simulink model "clutch_lockup"  (R2020b)
settings: Solver=VariableStepAuto  StartTime=0.0  StopTime=10.0  RelTol=1e-3
values from neighbouring files (symbols this model uses):
  be = 2.0    [initialization_data.sldd]
  bv = 1.0    [initialization_data.sldd]
  Ie = 1.0    [initialization_data.sldd]
  Iv = 5.0    [initialization_data.sldd]
  R = 1.0    [initialization_data.sldd]
  uk = 1.0    [initialization_data.sldd]
  us = 1.5    [initialization_data.sldd]
settings Model: Creator=Vrunda M Balgi  LastModifiedBy=Vrunda M Balgi

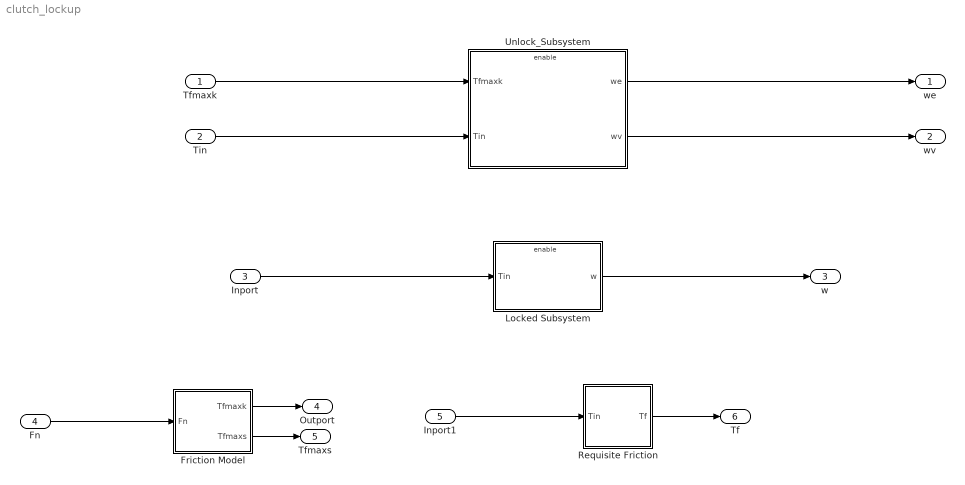
== system clutch_lockup ==
  Tfmaxk : Inport
  Tin : Inport  Port=2
  Inport : Inport  Port=3
  Fn : Inport  Port=4
  Inport1 : Inport  Port=5
  Friction Model : Subsystem
  Locked Subsystem : Subsystem
  Requisite Friction : Subsystem
  Unlock_Subsystem : Subsystem
  we : Outport
  wv : Outport  Port=2
  w : Outport  Port=3
  Outport : Outport  Port=4
  Tfmaxs : Outport  Port=5
  Tf : Outport  Port=6
  wires:
  Tfmaxk/1 -> Unlock_Subsystem/1(Tfmaxk)
  Tin/1 -> Unlock_Subsystem/2(Tin)
  Unlock_Subsystem/1(we) -> we/1
  Unlock_Subsystem/2(wv) -> wv/1
  Inport/1 -> Locked Subsystem/1(Tin)
  Locked Subsystem/1(w) -> w/1
  Fn/1 -> Friction Model/1(Fn)
  Friction Model/1(Tfmaxk) -> Outport/1
  Friction Model/2(Tfmaxs) -> Tfmaxs/1
  Inport1/1 -> Requisite Friction/1(Tin)
  Requisite Friction/1(Tf) -> Tf/1

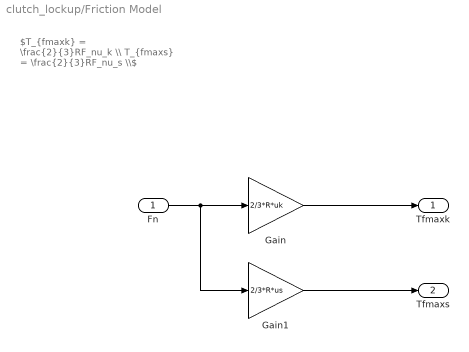
== system clutch_lockup/Friction Model ==
  note: $T_{fmaxk} = \frac{2}{3}RF_nu_k \\ T_{fmaxs} = \frac{2}{3}RF_nu_s \\$
  Fn : Inport
  Gain : Gain  Gain=2/3*R*uk
  Gain1 : Gain  Gain=2/3*R*us
  Tfmaxk : Outport
  Tfmaxs : Outport  Port=2
  wires:
  Gain1/1 -> Tfmaxs/1
  Fn/1 -> Gain1/1, Gain/1
  Gain/1 -> Tfmaxk/1

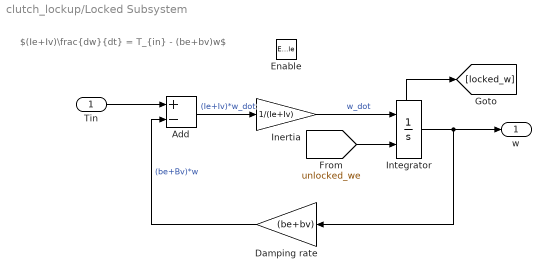
== system clutch_lockup/Locked Subsystem ==
  note: $(Ie+Iv)\frac{dw}{dt} = T_{in} - (be+bv)w$
  Tin : Inport
  Enable : EnablePort
  Add : Sum  Inputs=+-
  Damping rate : Gain  Gain=(be+bv)
  Inertia : Gain  Gain=1/(Ie+Iv)
  Integrator : Integrator  InitialConditionSource=external  ShowStatePort=on
  w : Outport
  wires:
  Inertia/1 -> Integrator/1  "w_dot"
  Add/1 -> Inertia/1  "(Ie+Iv)*w_dot"
  Tin/1 -> Add/1
  Integrator/State -> [locked_w]
  [unlocked_we] -> Integrator/2
  Integrator/1 -> w/1, Damping rate/1
  Damping rate/1 -> Add/2  "(be+Bv)*w"

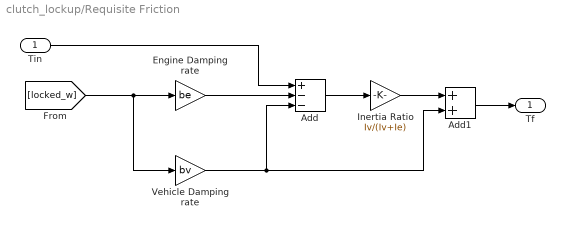
== system clutch_lockup/Requisite Friction ==
  Tin : Inport
  Add : Sum  Inputs=+--
  Add1 : Sum
  Engine Damping rate : Gain  Gain=be
  Inertia Ratio : Gain  Gain=Iv/(Iv+Ie)
  Vehicle Damping rate : Gain  Gain=bv
  Tf : Outport
  wires:
  [locked_w] -> Vehicle Damping rate/1, Engine Damping rate/1
  Vehicle Damping rate/1 -> Add1/2, Add/3
  Engine Damping rate/1 -> Add/2
  Add/1 -> Inertia Ratio/1
  Add1/1 -> Tf/1
  Inertia Ratio/1 -> Add1/1
  Tin/1 -> Add/1

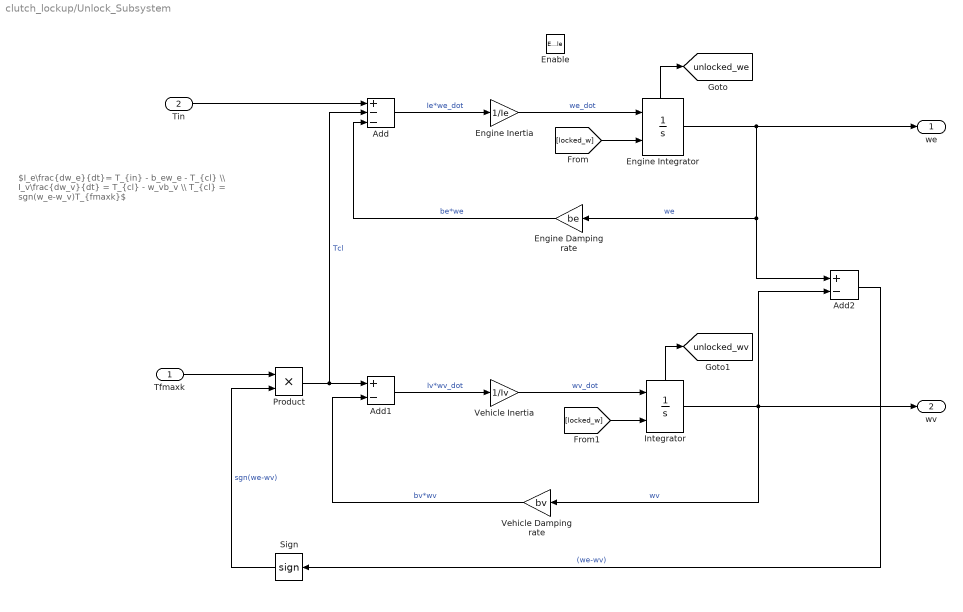
== system clutch_lockup/Unlock_Subsystem ==
  note: $I_e\frac{dw_e}{dt}= T_{in} - b_ew_e - T_{cl} \\ I_v\frac{dw_v}{dt} = T_{cl} - w_vb_v \\ T_{cl} = sgn(w_e-w_v)T_{fmaxk}$
  Tfmaxk : Inport
  Tin : Inport  Port=2
  Enable : EnablePort  StatesWhenEnabling=reset
  Add : Sum  Inputs=+--
  Add1 : Sum  Inputs=+-
  Add2 : Sum  Inputs=+-
  "Engine Damping rate " : Gain  Gain=be
  Engine Inertia : Gain  Gain=1/Ie
  Engine Integrator : Integrator  InitialConditionSource=external  ShowStatePort=on
  Integrator : Integrator  InitialConditionSource=external  ShowStatePort=on
  Product : Product
  Sign : Signum
  Vehicle Damping rate : Gain  Gain=bv
  Vehicle Inertia : Gain  Gain=1/Iv
  we : Outport
  wv : Outport  Port=2
  tag scope: unlocked_we=global, unlocked_wv=global
  wires:
  Integrator/State -> [unlocked_wv]
  Engine Integrator/1 -> we/1, Add2/1, "Engine Damping rate "/1  "we"
  Integrator/1 -> wv/1, Add2/2, Vehicle Damping rate/1  "wv"
  [locked_w] -> Integrator/2
  Add1/1 -> Vehicle Inertia/1  "Iv*wv_dot"
  Add/1 -> Engine Inertia/1  "Ie*we_dot"
  Vehicle Inertia/1 -> Integrator/1  "wv_dot"
  Sign/1 -> Product/2  "sgn(we-wv)"
  Engine Inertia/1 -> Engine Integrator/1  "we_dot"
  Product/1 -> Add/2, Add1/1  "Tcl"
  Tin/1 -> Add/1
  Add2/1 -> Sign/1  "(we-wv)"
  [locked_w] -> Engine Integrator/2
  Engine Integrator/State -> [unlocked_we]
  "Engine Damping rate "/1 -> Add/3  "be*we"
  Tfmaxk/1 -> Product/1
  Vehicle Damping rate/1 -> Add1/2  "bv*wv"
